simulink model "PWM"  (R2023b)
settings: Solver=VariableStepAuto  StartTime=0.0  StopTime=0.02  RelTol=1e-3
libraries: simulink x1, spsTriangleGeneratorLib x1
settings Model: Creator=Ketan  LastModifiedBy=HP5CD

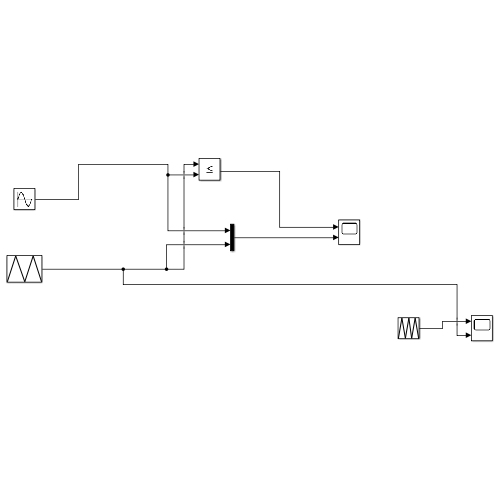
[thumbnail: Simulink's stored preview of the top-level diagram]
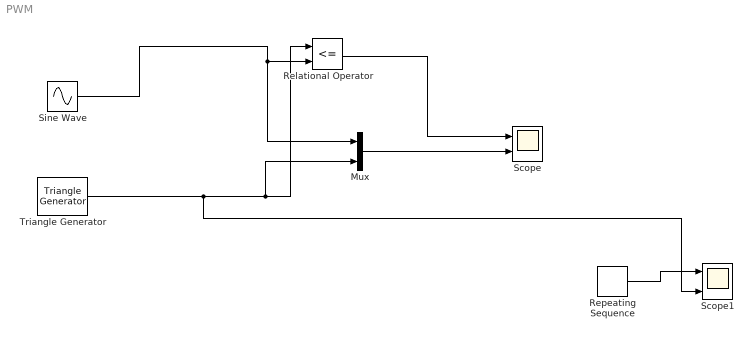
== system PWM ==
  Mux : Mux  Inputs=2
  Relational Operator : RelationalOperator  Operator=<=  OutDataTypeStr=boolean  RndMeth=Simplest  InputSameDT=off
  Repeating Sequence : simulink/Sources/Repeating Sequence  rep_seq_t=[0 5e-4 1e-3]  rep_seq_y=[-1 1 -1]
  Scope : Scope  NumInputPorts=2
  Scope1 : Scope  NumInputPorts=2
  Sine Wave : Sin  Amplitude=0.9  Frequency=2*pi*50  SampleTime=0
  Triangle Generator : spsTriangleGeneratorLib/Triangle Generator  Freq=1e3  Phase=0  Ts=0
  wires:
  Sine Wave/1 -> Relational Operator/2, Mux/1
  Relational Operator/1 -> Scope/1
  Mux/1 -> Scope/2
  Triangle Generator/1 -> Scope1/2, Relational Operator/1, Mux/2
  Repeating Sequence/1 -> Scope1/1
